simulink model "modification_consigne_copy"  (R2019b)
settings: Solver=FixedStepAuto  StartTime=0.0  StopTime=inf  FixedStep=0.01  RelTol=1e-3  EnableMultiTasking=on
libraries: arduinolib x13, dspstat3 x5, simulink x2, LCDlib x1, Laboratoire x1
settings Model: SILPILModeSetting=veronly  ExtModeTrigDuration=2  Creator=Etudiant  LastModifiedBy=Etudiant
settings OptimizationCC: EnhancedBackFolding=on  PassReuseOutputArgsAs=Individual arguments  ZeroExternalMemoryAtStartup=off  ZeroInternalMemoryAtStartup=off  MaxStackSize=64  OptimizeBlockOrder=speed  DifferentSizesBufferReuse=on  OptimizationCustomize=off  EfficientTunableParamExpr=on
settings DebuggingCC: ParameterTunabilityLossMsg=error
settings HardwareCC: ProdBitPerInt=16  ProdBitPerPointer=16  ProdBitPerSizeT=16  ProdBitPerPtrDiffT=16  ProdLargestAtomicFloat=None  ProdWordSize=8  ProdHWDeviceType=Atmel->AVR
settings SFSimCC: MATLABDynamicMemAlloc=off
settings RTWCC: SystemTargetFile=ert.tlc  HardwareBoard=Arduino Mega 2560  TLCOptions=-aInlineSetEventsForThisBaseRateFcn=TLC_FALSE -aSuppressMultiTaskScheduler=TLC_FALSE -aRateBasedStepFcn=1  TemplateMakefile=ert_default_tmf  CustomSource=enc_eml_src.c  Toolchain=Arduino AVR  BuildConfiguration=Faster Runs  IncludeHyperlinkInReport=on
settings CodeAppCC: ForceParamTrailComments=on  GenerateComments=off  IgnoreCustomStorageClasses=off  OperatorAnnotations=on  SimulinkDataObjDesc=on  SFDataObjDesc=on  InsertBlockDesc=on
settings ERTTargetCC: SupportContinuousTime=on  SupportVariableSizeSignals=on  ExtModeStaticAllocSize=2048

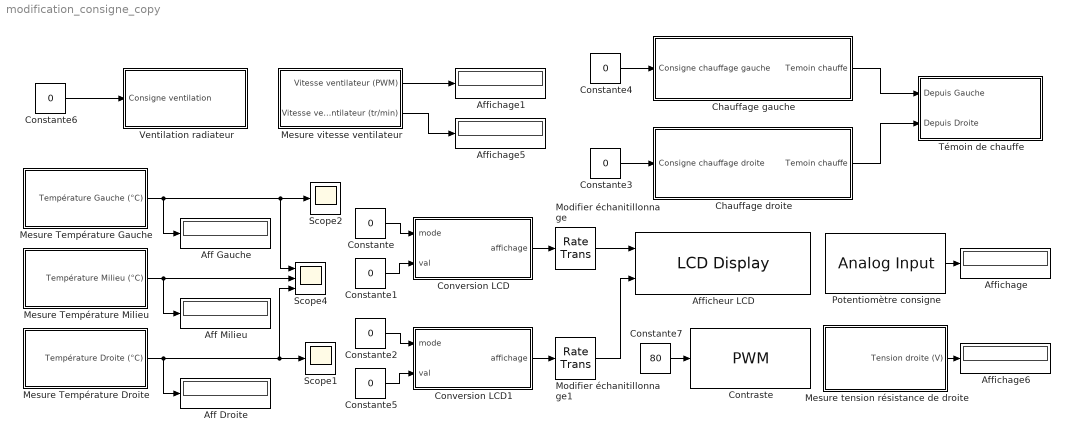
== system modification_consigne_copy ==
  Aff Droite : Display
  Aff Gauche : Display
  Aff Milieu : Display
  Affichage{,1,5..6} (4 alike) : Display
  Afficheur LCD : LCDlib/LCD Display  pins=[30, 31, 32, 34, 36, 38]
      settings: SourceProductName=Arduino Extra Library
  Chauffage droite : Subsystem
  Chauffage gauche : Subsystem
  Constante : Constant  Value=0  OutDataTypeStr=uint8  SampleTime=-1
  Constante{1,3..6} (5 alike) : Constant  Value=0  SampleTime=-1
  Constante2 : Constant  Value=0  OutDataTypeStr=uint8  SampleTime=-1
  Constante7 : Constant  Value=80  SampleTime=-1
  Contraste : arduinolib/PWM  pinNumber=44  EnableInputFrequency=off  InitialFrequency=2000  InitialDutyCycle=0  NotificationType=None  blockPlatform=arduino
  Conversion LCD : MATLAB Function  TreatAsAtomicUnit=on
  Conversion LCD1 : MATLAB Function  TreatAsAtomicUnit=on
  Mesure Température Droite : Subsystem
  Mesure Température Gauche : Subsystem
  Mesure Température Milieu : Subsystem
  Mesure tension résistance de droite : Subsystem
  Mesure vitesse ventilateur : Subsystem
  Modifier échanitillonnage : RateTransition  Integrity=off  OutPortSampleTime=1
  Modifier échanitillonnage1 : RateTransition  Integrity=off  OutPortSampleTime=1
  Potentiomètre consigne : arduinolib/Analog Input  pinNumber=3  ReadResultsOnly=off  ConversionTriggerSource=Software  ExternalTriggerType=uint32(0)  OutputDataType=uint16  EnableConversionCompleteNotify=off  EnableOuputStatus=off  SampleTime=-1  blockPlatform=arduino
  Scope1 : Scope
  Scope2 : Scope
  Scope4 : Scope  NumInputPorts=3
  Témoin de chauffe : Subsystem
  Ventilation radiateur : Subsystem
  wires:
  Potentiomètre consigne/1 -> Affichage/1
  Mesure tension résistance de droite/1(Tension droite (V)) -> Affichage6/1
  Constante3/1 -> Chauffage droite/1(Consigne chauffage droite)
  Constante4/1 -> Chauffage gauche/1(Consigne chauffage gauche)
  Constante6/1 -> Ventilation radiateur/1(Consigne ventilation)
  Mesure vitesse ventilateur/1(Vitesse ventilateur (PWM)) -> Affichage1/1
  Mesure vitesse ventilateur/2(Vitesse ventilateur (tr/min)) -> Affichage5/1
  Chauffage gauche/1(Temoin chauffe) -> Témoin de chauffe/1(Depuis Gauche)
  Chauffage droite/1(Temoin chauffe) -> Témoin de chauffe/2(Depuis Droite)
  Mesure Température Gauche/1(Température Gauche (°C)) -> Scope2/1, Scope4/1, Aff Gauche/1
  Mesure Température Milieu/1(Température Milieu (°C)) -> Scope4/2, Aff Milieu/1
  Mesure Température Droite/1(Température Droite (°C)) -> Scope4/3, Scope1/1, Aff Droite/1
  Conversion LCD/1(affichage) -> Modifier échanitillonnage/1
  Constante/1 -> Conversion LCD/1(mode)
  Constante1/1 -> Conversion LCD/2(val)
  Constante7/1 -> Contraste/1
  Constante2/1 -> Conversion LCD1/1(mode)
  Constante5/1 -> Conversion LCD1/2(val)
  Conversion LCD1/1(affichage) -> Modifier échanitillonnage1/1
  Modifier échanitillonnage/1 -> Afficheur LCD/1
  Modifier échanitillonnage1/1 -> Afficheur LCD/2

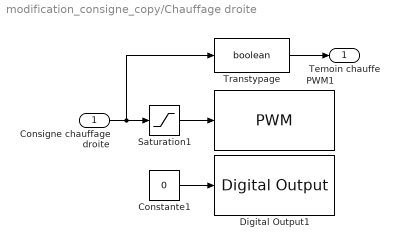
== system modification_consigne_copy/Chauffage droite ==
  Consigne chauffage droite : Inport
  Constante1 : Constant  Value=0  SampleTime=-1
  Digital Output1 : arduinolib/Digital Output  pinNumber=10  blockPlatform=arduino
  PWM1 : arduinolib/PWM  pinNumber=7  EnableInputFrequency=off  InitialFrequency=2000  InitialDutyCycle=0  NotificationType=None  blockPlatform=arduino
  Saturation1 : Saturate  UpperLimit=255  LowerLimit=0
  Transtypage : DataTypeConversion  OutDataTypeStr=boolean
  Temoin chauffe : Outport  VectorParamsAs1DForOutWhenUnconnected=off
  wires:
  Saturation1/1 -> PWM1/1
  Constante1/1 -> Digital Output1/1
  Consigne chauffage droite/1 -> Transtypage/1, Saturation1/1
  Transtypage/1 -> Temoin chauffe/1

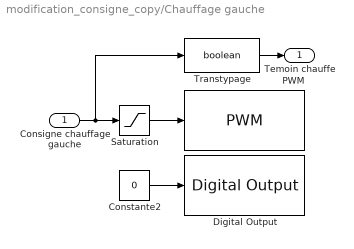
== system modification_consigne_copy/Chauffage gauche ==
  Consigne chauffage gauche : Inport
  Constante2 : Constant  Value=0  SampleTime=-1
  Digital Output : arduinolib/Digital Output  pinNumber=9  blockPlatform=arduino
  PWM : arduinolib/PWM  pinNumber=6  EnableInputFrequency=off  InitialFrequency=2000  InitialDutyCycle=0  NotificationType=None  blockPlatform=arduino
  Saturation : Saturate  UpperLimit=255  LowerLimit=0
  Transtypage : DataTypeConversion  OutDataTypeStr=boolean
  Temoin chauffe : Outport  VectorParamsAs1DForOutWhenUnconnected=off
  wires:
  Constante2/1 -> Digital Output/1
  Saturation/1 -> PWM/1
  Consigne chauffage gauche/1 -> Transtypage/1, Saturation/1
  Transtypage/1 -> Temoin chauffe/1

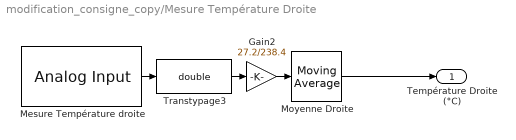
== system modification_consigne_copy/Mesure Température Droite ==
  Gain2 : Gain  Gain=27.2/238.4
  Mesure Température droite : arduinolib/Analog Input  pinNumber=2  ReadResultsOnly=off  ConversionTriggerSource=Software  ExternalTriggerType=uint32(0)  OutputDataType=uint16  EnableConversionCompleteNotify=off  EnableOuputStatus=off  SampleTime=-1  blockPlatform=arduino
  Moyenne Droite : dspstat3/Moving Average  Method=Sliding window  ForgettingFactorPort=off  SpecifyWindowLength=on  WindowLength=5  ForgettingFactor=0.9  SimulateUsing=Code generation
  Transtypage3 : DataTypeConversion  OutDataTypeStr=double
  Température Droite (°C) : Outport
  wires:
  Gain2/1 -> Moyenne Droite/1
  Moyenne Droite/1 -> Température Droite (°C)/1
  Mesure Température droite/1 -> Transtypage3/1
  Transtypage3/1 -> Gain2/1

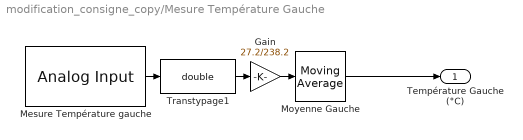
== system modification_consigne_copy/Mesure Température Gauche ==
  Gain : Gain  Gain=27.2/238.2
  Mesure Température gauche : arduinolib/Analog Input  pinNumber=0  ReadResultsOnly=off  ConversionTriggerSource=Software  ExternalTriggerType=uint32(0)  OutputDataType=uint16  EnableConversionCompleteNotify=off  EnableOuputStatus=off  SampleTime=-1  blockPlatform=arduino
  Moyenne Gauche : dspstat3/Moving Average  Method=Sliding window  ForgettingFactorPort=off  SpecifyWindowLength=on  WindowLength=5  ForgettingFactor=0.9  SimulateUsing=Code generation
  Transtypage1 : DataTypeConversion  OutDataTypeStr=double
  Température Gauche (°C) : Outport
  wires:
  Gain/1 -> Moyenne Gauche/1
  Mesure Température gauche/1 -> Transtypage1/1
  Transtypage1/1 -> Gain/1
  Moyenne Gauche/1 -> Température Gauche (°C)/1

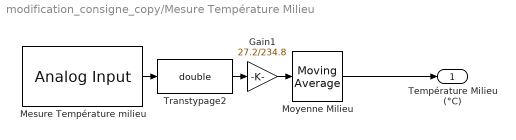
== system modification_consigne_copy/Mesure Température Milieu ==
  Gain1 : Gain  Gain=27.2/234.8
  Mesure Température milieu : arduinolib/Analog Input  pinNumber=1  ReadResultsOnly=off  ConversionTriggerSource=Software  ExternalTriggerType=uint32(0)  OutputDataType=uint16  EnableConversionCompleteNotify=off  EnableOuputStatus=off  SampleTime=-1  blockPlatform=arduino
  Moyenne Milieu : dspstat3/Moving Average  Method=Sliding window  ForgettingFactorPort=off  SpecifyWindowLength=on  WindowLength=5  ForgettingFactor=0.9  SimulateUsing=Code generation
  Transtypage2 : DataTypeConversion  OutDataTypeStr=double
  Température Milieu (°C) : Outport
  wires:
  Gain1/1 -> Moyenne Milieu/1
  Mesure Température milieu/1 -> Transtypage2/1
  Transtypage2/1 -> Gain1/1
  Moyenne Milieu/1 -> Température Milieu (°C)/1

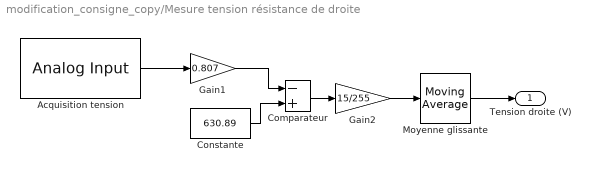
== system modification_consigne_copy/Mesure tension résistance de droite ==
  Acquisition tension : arduinolib/Analog Input  pinNumber=4  ReadResultsOnly=off  ConversionTriggerSource=Software  ExternalTriggerType=uint32(0)  OutputDataType=uint16  EnableConversionCompleteNotify=off  EnableOuputStatus=off  SampleTime=-1  blockPlatform=arduino
  Comparateur : Sum  Inputs=-+  OutDataTypeStr=double
  Constante : Constant  Value=630.89  SampleTime=-1
  Gain1 : Gain  Gain=0.807
  Gain2 : Gain  Gain=15/255
  Moyenne glissante : dspstat3/Moving Average  Method=Sliding window  ForgettingFactorPort=off  SpecifyWindowLength=on  WindowLength=4  ForgettingFactor=0.9  SimulateUsing=Code generation
  Tension droite (V) : Outport
  wires:
  Acquisition tension/1 -> Gain1/1
  Gain2/1 -> Moyenne glissante/1
  Constante/1 -> Comparateur/2
  Comparateur/1 -> Gain2/1
  Moyenne glissante/1 -> Tension droite (V)/1
  Gain1/1 -> Comparateur/1

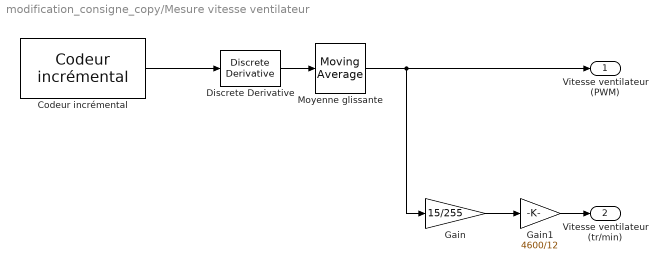
== system modification_consigne_copy/Mesure vitesse ventilateur ==
  Codeur incrémental : Laboratoire/Arduino/Codeur incrémental  enc=0  pinA=2  pinB=2  T=-1
      settings: SourceProductName=Laboratoire Dautet
  Discrete Derivative : simulink/Discrete/Discrete Derivative  gainval=1.0  ICPrevScaledInput=0.0  OutMin=[]  OutMax=[]  OutDataType=fixdt(1, 16)  OutScaling=2^-10  DoSatur=off
  Gain : Gain  Gain=15/255
  Gain1 : Gain  Gain=4600/12
  Moyenne glissante : dspstat3/Moving Average  Method=Sliding window  ForgettingFactorPort=off  SpecifyWindowLength=on  WindowLength=5  ForgettingFactor=0.9  SimulateUsing=Code generation
  Vitesse ventilateur (PWM) : Outport
  Vitesse ventilateur (tr/min) : Outport  Port=2
  wires:
  Discrete Derivative/1 -> Moyenne glissante/1
  Moyenne glissante/1 -> Vitesse ventilateur (PWM)/1, Gain/1
  Codeur incrémental/1 -> Discrete Derivative/1
  Gain/1 -> Gain1/1
  Gain1/1 -> Vitesse ventilateur (tr/min)/1

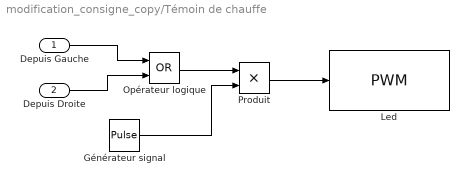
== system modification_consigne_copy/Témoin de chauffe ==
  Depuis Gauche : Inport
  Depuis Droite : Inport  Port=2
  Générateur signal : DiscretePulseGenerator  PulseType=Time based  Amplitude=255  PulseWidth=50
  Led : arduinolib/PWM  pinNumber=11  EnableInputFrequency=off  InitialFrequency=2000  InitialDutyCycle=0  NotificationType=None  blockPlatform=arduino
  Opérateur logique : Logic  Operator=OR  AllPortsSameDT=off  OutDataTypeStr=boolean
  Produit : Product
  wires:
  Depuis Gauche/1 -> Opérateur logique/1
  Depuis Droite/1 -> Opérateur logique/2
  Opérateur logique/1 -> Produit/1
  Générateur signal/1 -> Produit/2
  Produit/1 -> Led/1

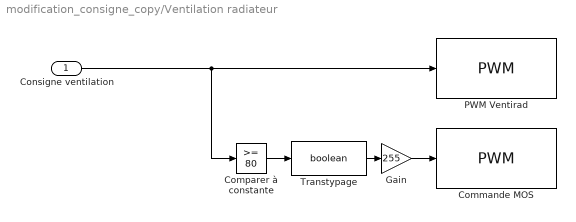
== system modification_consigne_copy/Ventilation radiateur ==
  Consigne ventilation : Inport
  Commande MOS : arduinolib/PWM  pinNumber=8  EnableInputFrequency=off  InitialFrequency=2000  InitialDutyCycle=0  NotificationType=None  blockPlatform=arduino
  Comparer à constante : simulink/Logic and Bit Operations/Compare To Constant  relop=>=  const=80  OutDataTypeStr=boolean
  Gain : Gain  Gain=255
  PWM Ventirad : arduinolib/PWM  pinNumber=12  EnableInputFrequency=off  InitialFrequency=2000  InitialDutyCycle=0  NotificationType=None  blockPlatform=arduino
  Transtypage : DataTypeConversion  OutDataTypeStr=boolean
  wires:
  Consigne ventilation/1 -> Comparer à constante/1, PWM Ventirad/1
  Transtypage/1 -> Gain/1
  Gain/1 -> Commande MOS/1
  Comparer à constante/1 -> Transtypage/1

== matlab function modification_consigne_copy/Conversion LCD1 ==
  data: mode input uint8; val input size=1; affichage output uint8 size=1 16
function affichage = fcn(mode, val)

% Guy Labasse - Lycée Dautet 2019
% Modifié pour TP Régulation CPU

% mode == 0 --> Test Afficheur
% mode == 1 --> température
% mode == 2 --> 
% mode == 3 --> 
% mode == 4 --> 
% mode == 5 --> 
% mode == 6 --> 
% mode == 7 --> Bienvenue ...
% Toute autre valeur de mode --> Erreur !

% val: valeur numérique réel double précision

% La fonction décode de 000 à 999
% Toute valeur au delà sera saturée à 999

affichage           = uint8(zeros([1 16]));
valeur              = single(val);
mode                = uint8(mode);


%% Affichage sur trois caractères

% Premier caratère (centaines)
v           = fix(valeur);
a           = abs(v);

if a>=0 && a<100
    affichage(9)    = uint8(48);
    b       = a;
    
elseif a>=100 && a<200
    affichage(9)    = uint8(49);
    b       = a-100;
    
elseif a>=200 && a<300
    affichage(9)    = uint8(50);
    b       = a-200;
    
elseif a>=300 && a<400
    affichage(9)    = uint8(51);
    b       = a-300;
    
elseif a>=400 && a<500
    affichage(9)    = uint8(52);
    b       = a-400;
    
elseif a>=500 && a<600
    affichage(9)    = uint8(53);
    b       = a-500;
    
elseif a>=600 && a<700
    affichage(9)    = uint8(54);
    b       = a-600;
    
elseif a>=700 && a<800
    affichage(9)    = uint8(55);
    b       = a-700;
    
elseif a>=800 && a<900
    affichage(9)    = uint8(56);
    b       = a-800;
    
elseif a>=900 && a<1000
    affichage(9)    = uint8(57);
    b       = a-900;
    
else
    affichage(9)    = uint8(57);
    b       = single(99);
end

% Deuxième caratère (dizaines)

if b>=0 && b<10
    affichage(10)    = uint8(48);
    c       = b;
    
elseif b>=10 && b<20
    affichage(10)    = uint8(49);
    c       = b-10;
    
elseif b>=20 && b<30
    affichage(10)    = uint8(50);
    c       = b-20;
    
elseif b>=30 && b<40
    affichage(10)    = uint8(51);
    c       = b-30;
    
elseif b>=40 && b<50
    affichage(10)    = uint8(52);
    c       = b-40;
    
elseif b>=50 && b<60
    affichage(10)    = uint8(53);
    c       = b-50;
    
elseif b>=60 && b<70
    affichage(10)    = uint8(54);
    c       = b-60;
    
elseif b>=70 && b<80
    affichage(10)    = uint8(55);
    c       = b-70;
    
elseif b>=80 && b<90
    affichage(10)    = uint8(56);
    c       = b-80;
    
elseif b>=90 && b<100
    affichage(10)    = uint8(57);
    c       = b-90;
    
else
    affichage(10)    = uint8(57);
    c       = single(9);
end

% Troisième caratère (unités)
affichage(11)        = determineNombre(c);

%% Gestion du mode d'affichage
if mode == 0
    affichage(1:16)      = uint8([84 101 115 116 32 97 102 102 105 99 104 101 117 114 32 32]);
elseif mode == 1
    affichage(1:7)      = uint8([84   101   109   112    58    32   32]);
    affichage([14 15 16])  = uint8([32 67 32]);
elseif mode == 2
    affichage(1:7)      = uint8([72   117   109   105    58    32   32]);
    affichage([14 15 16])  = uint8([32 37 32]);
elseif mode == 3
    affichage(1:7)      = uint8([77   97   115   115    101    58   32]);
    affichage([14 15 16])  = uint8([32 103 32]);
elseif mode == 4
    affichage(1:7)      = uint8([86   111   108   117    109    101   58]);
    affichage([14 15 16])  = uint8([32 109 108]);
elseif mode == 5
    affichage(1:16)      = uint8([84 80 32 66 97 108 97 110 99 101 32 72 97 108 111 32]);
elseif mode == 6
    affichage(1:16)      = uint8([45 45 45 45 32 32 32 32 32 32 32 32 32 32 32 32]);
elseif mode == 7
    affichage(1:16)      = uint8([66 105 101 110 118 101 110 117 101 32 46 46 46 32 32 32]);
else
    affichage(1:16)      = uint8([69 114 114 101 117 114 32 33 32 32 32 32 32 32 32 32]);
end

end


%% Affichage Ascii des caractères

function d = determineNombre(n)

    switch n
        case 0
            d = uint8(48);
        case 1
            d = uint8(49);
        case 2
            d = uint8(50);
        case 3
            d = uint8(51);
        case 4
            d = uint8(52);
        case 5
            d = uint8(53);
        case 6
            d = uint8(54);
        case 7
            d = uint8(55);
        case 8
            d = uint8(56);
        case 9
            d = uint8(57);    
        otherwise
            d = uint8(57);
    end

end

== matlab function modification_consigne_copy/Conversion LCD ==
  data: mode input uint8; val input size=1; affichage output uint8 size=1 16
function affichage = fcn(mode, val)

% Guy Labasse - Lycée Dautet 2019
% Modifié pour TP Régulation CPU

% mode == 0 --> Test Afficheur
% mode == 1 --> température
% mode == 2 --> 
% mode == 3 --> 
% mode == 4 --> 
% mode == 5 --> 
% mode == 6 --> 
% mode == 7 --> Bienvenue ...
% Toute autre valeur de mode --> Erreur !

% val: valeur numérique réel double précision

% La fonction décode de 000 à 999
% Toute valeur au delà sera saturée à 999

affichage           = uint8(zeros([1 16]));
valeur              = single(val);
mode                = uint8(mode);


%% Affichage sur trois caractères

% Premier caratère (centaines)
v           = fix(valeur);
a           = abs(v);

if a>=0 && a<100
    affichage(9)    = uint8(48);
    b       = a;
    
elseif a>=100 && a<200
    affichage(9)    = uint8(49);
    b       = a-100;
    
elseif a>=200 && a<300
    affichage(9)    = uint8(50);
    b       = a-200;
    
elseif a>=300 && a<400
    affichage(9)    = uint8(51);
    b       = a-300;
    
elseif a>=400 && a<500
    affichage(9)    = uint8(52);
    b       = a-400;
    
elseif a>=500 && a<600
    affichage(9)    = uint8(53);
    b       = a-500;
    
elseif a>=600 && a<700
    affichage(9)    = uint8(54);
    b       = a-600;
    
elseif a>=700 && a<800
    affichage(9)    = uint8(55);
    b       = a-700;
    
elseif a>=800 && a<900
    affichage(9)    = uint8(56);
    b       = a-800;
    
elseif a>=900 && a<1000
    affichage(9)    = uint8(57);
    b       = a-900;
    
else
    affichage(9)    = uint8(57);
    b       = single(99);
end

% Deuxième caratère (dizaines)

if b>=0 && b<10
    affichage(10)    = uint8(48);
    c       = b;
    
elseif b>=10 && b<20
    affichage(10)    = uint8(49);
    c       = b-10;
    
elseif b>=20 && b<30
    affichage(10)    = uint8(50);
    c       = b-20;
    
elseif b>=30 && b<40
    affichage(10)    = uint8(51);
    c       = b-30;
    
elseif b>=40 && b<50
    affichage(10)    = uint8(52);
    c       = b-40;
    
elseif b>=50 && b<60
    affichage(10)    = uint8(53);
    c       = b-50;
    
elseif b>=60 && b<70
    affichage(10)    = uint8(54);
    c       = b-60;
    
elseif b>=70 && b<80
    affichage(10)    = uint8(55);
    c       = b-70;
    
elseif b>=80 && b<90
    affichage(10)    = uint8(56);
    c       = b-80;
    
elseif b>=90 && b<100
    affichage(10)    = uint8(57);
    c       = b-90;
    
else
    affichage(10)    = uint8(57);
    c       = single(9);
end

% Troisième caratère (unités)
affichage(11)        = determineNombre(c);

%% Gestion du mode d'affichage
if mode == 0
    affichage(1:16)      = uint8([84 101 115 116 32 97 102 102 105 99 104 101 117 114 32 32]);
elseif mode == 1
    affichage(1:7)      = uint8([84   101   109   112    58    32   32]);
    affichage([14 15 16])  = uint8([32 67 32]);
elseif mode == 2
    affichage(1:7)      = uint8([72   117   109   105    58    32   32]);
    affichage([14 15 16])  = uint8([32 37 32]);
elseif mode == 3
    affichage(1:7)      = uint8([77   97   115   115    101    58   32]);
    affichage([14 15 16])  = uint8([32 103 32]);
elseif mode == 4
    affichage(1:7)      = uint8([86   111   108   117    109    101   58]);
    affichage([14 15 16])  = uint8([32 109 108]);
elseif mode == 5
    affichage(1:16)      = uint8([84 80 32 66 97 108 97 110 99 101 32 72 97 108 111 32]);
elseif mode == 6
    affichage(1:16)      = uint8([45 45 45 45 32 32 32 32 32 32 32 32 32 32 32 32]);
elseif mode == 7
    affichage(1:16)      = uint8([66 105 101 110 118 101 110 117 101 32 46 46 46 32 32 32]);
else
    affichage(1:16)      = uint8([69 114 114 101 117 114 32 33 32 32 32 32 32 32 32 32]);
end

end


%% Affichage Ascii des caractères

function d = determineNombre(n)

    switch n
        case 0
            d = uint8(48);
        case 1
            d = uint8(49);
        case 2
            d = uint8(50);
        case 3
            d = uint8(51);
        case 4
            d = uint8(52);
        case 5
            d = uint8(53);
        case 6
            d = uint8(54);
        case 7
            d = uint8(55);
        case 8
            d = uint8(56);
        case 9
            d = uint8(57);    
        otherwise
            d = uint8(57);
    end

end
